simulink model "step_response"  (R2020b)
settings: Solver=VariableStepAuto  StartTime=0.0  StopTime=10.0  RelTol=1e-3
model workspace: external: MATLAB File C:\Users\deves\MATLAB\Projects\problem5\data5.m (data not in the file)
values from neighbouring files (symbols this model uses):
  C = 10    [data5.m]
  R = 10    [data5.m]
settings Model: Creator=deves  LastModifiedBy=deves

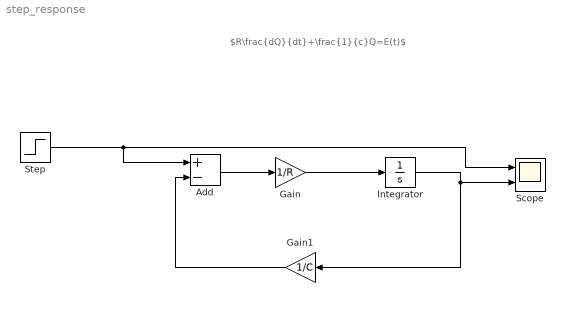
== system step_response ==
  note: $R\frac{dQ}{dt}+\frac{1}{c}Q=E(t)$
  Add : Sum  Inputs=+-
  Gain : Gain  Gain=1/R
  Gain1 : Gain  Gain=1/C
  Integrator : Integrator  InitialCondition=0.5
  Scope : Scope  NumInputPorts=2
  Step : Step  SampleTime=0
  wires:
  Gain/1 -> Integrator/1
  Add/1 -> Gain/1
  Integrator/1 -> Gain1/1, Scope/2
  Gain1/1 -> Add/2
  Step/1 -> Scope/1, Add/1
